simulink model "pondera2"  (R2020b)
settings: Solver=ode5  StartTime=0.0  StopTime=inf  RelTol=1e-3
undefined symbols (not defined in the file): National_Instruments, PCI
libraries: sldrtlib x2
settings Model: SimulationMode=external  Creator=Usuario_UMA  LastModifiedBy=alumnoic03
settings RTWCC: Description=Simulink Desktop Real-Time  SystemTargetFile=sldrt.tlc  TemplateMakefile=sldrt.tmf  RTWCompilerOptimization=on
settings CodeAppCC: MaxIdLength=95
settings SimulinkDesktopRealTimeCC: TargetPreCompLibLocation=C:\Program Files\MATLAB\R2020\toolbox\sldrt\lib\win64

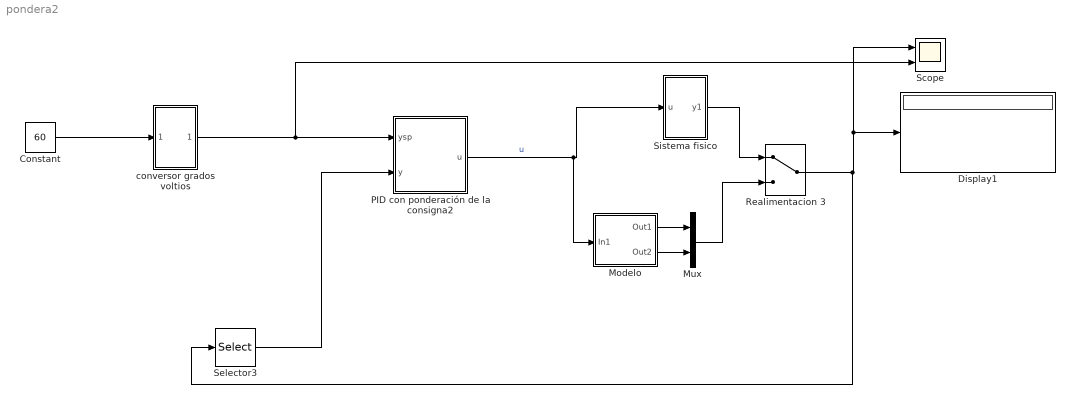
== system pondera2 ==
  Constant : Constant  Value=60
  Display1 : Display
  "Modelo " : Subsystem
  Mux : Mux  Inputs=2
  PID con ponderación de la consigna2 : Subsystem  mask{Kp=1.96, Ti=1.17, Td=0.118, b=0.85, c=0.1, N=30}
      mask prompts: Kp "Ganancia Proporcional (Kp)"; Ti "Tiempo Integral (Ti) [s]"; Td "Tiempo Derivativo (Td) [s]"; b "Peso Error Proporcional (b)"; c "Peso Error Derivativo (c)"; N "Filtro Derivativo (N) [rad/s]"
  Realimentacion 3 : ManualSwitch
  Scope : Scope  NumInputPorts=2
  Selector3 : Selector  InputPortWidth=2  IndexOptions=Index vector (dialog)  Indices=[1]  OutputSizes=1
  Sistema fisico : Subsystem
  "conversor grados voltios " : Subsystem  mask{a=4.95, b=0}
  wires:
  Constant/1 -> "conversor grados voltios "/1(In1)
  "conversor grados voltios "/1(Out1) -> PID con ponderación de la consigna2/1(ysp), Scope/2
  Selector3/1 -> PID con ponderación de la consigna2/2(y)
  PID con ponderación de la consigna2/1(u) -> "Modelo "/1(In1), Sistema fisico/1(u)  "u"
  "Modelo "/2(Out2) -> Mux/2
  "Modelo "/1(Out1) -> Mux/1
  Sistema fisico/1(y1) -> Realimentacion 3/1
  Mux/1 -> Realimentacion 3/2
  Realimentacion 3/1 -> Selector3/1, Display1/1, Scope/1

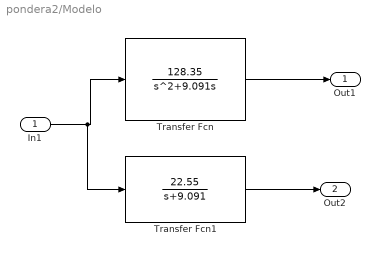
== system pondera2/Modelo  ==
  In1 : Inport
  Transfer Fcn : TransferFcn  Numerator=[128.35]  Denominator=[1 9.091 0]
  Transfer Fcn1 : TransferFcn  Numerator=[22.55]  Denominator=[1 9.091]
  Out1 : Outport
  Out2 : Outport  Port=2
  wires:
  In1/1 -> Transfer Fcn1/1, Transfer Fcn/1
  Transfer Fcn/1 -> Out1/1
  Transfer Fcn1/1 -> Out2/1

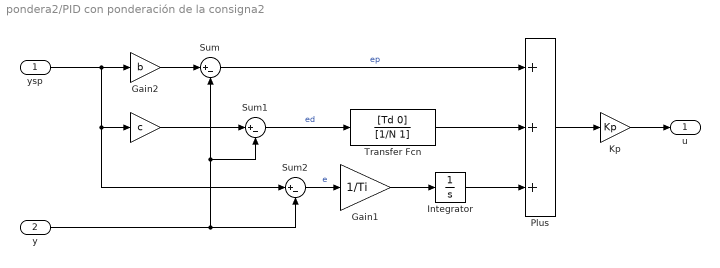
== system pondera2/PID con ponderación de la consigna2 ==
  ysp : Inport
  y : Inport  Port=2
  " " : Gain  Gain=c
  Gain1 : Gain  Gain=1/Ti
  Gain2 : Gain  Gain=b
  Integrator : Integrator
  Kp : Gain  Gain=Kp
  Plus : Sum  Inputs=+++
  Sum : Sum  Inputs=|+-
  Sum1 : Sum  Inputs=|+-
  Sum2 : Sum  Inputs=|+-
  Transfer Fcn : TransferFcn  Numerator=[Td 0]  Denominator=[1/N 1]
  u : Outport  VectorParamsAs1DForOutWhenUnconnected=off
  wires:
  Plus/1 -> Kp/1
  Kp/1 -> u/1
  Gain1/1 -> Integrator/1
  Integrator/1 -> Plus/3
  Transfer Fcn/1 -> Plus/2
  ysp/1 -> Sum2/1, " "/1, Gain2/1
  Gain2/1 -> Sum/1
  Sum/1 -> Plus/1  "ep"
  " "/1 -> Sum1/1
  Sum2/1 -> Gain1/1  "e"
  Sum1/1 -> Transfer Fcn/1  "ed"
  y/1 -> Sum/2, Sum1/2, Sum2/2

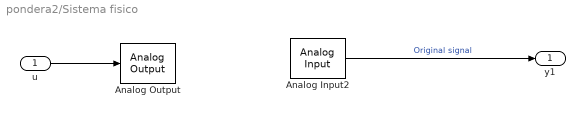
== system pondera2/Sistema fisico ==
  u : Inport
  Analog Input2 : sldrtlib/Analog Input  SampleTime=0.001  MaxMissedTicks=10  ShowMissedTicks=off  YieldWhenWaiting=off  DrvName=National_Instruments/PCI-6014  DrvAddress=4294967295  DrvOptions=[2 0 0 0 0 0]  Channels=[1,2]  RangeMode=1  VoltRange=1  DataType=1
      settings: AttributesFormatString=National Instruments\nPCI-6014 [auto]
  Analog Output : sldrtlib/Analog Output  SampleTime=0.001  MaxMissedTicks=10  ShowMissedTicks=off  YieldWhenWaiting=off  DrvName=National_Instruments/PCI-6014  DrvAddress=4294967295  DrvOptions=[2 0 0 0 0 0]  Channels=1  RangeMode=1  VoltRange=1  InitialValue=[]  FinalValue=[]
      settings: AttributesFormatString=National Instruments\nPCI-6014 [auto]
  y1 : Outport
  wires:
  u/1 -> Analog Output/1
  Analog Input2/1 -> y1/1  "Original signal"

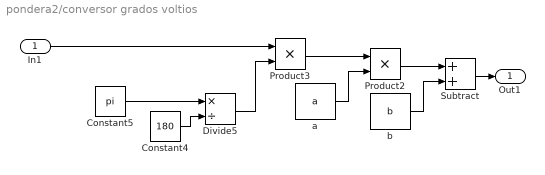
== system pondera2/conversor grados voltios  ==
  In1 : Inport
  Constant4 : Constant  Value=180
  Constant5 : Constant  Value=pi
  Divide5 : Product  Inputs=*/
  Product2 : Product
  Product3 : Product
  Subtract : Sum
  a : Constant  Value=a
  b : Constant  Value=b
  Out1 : Outport
  wires:
  b/1 -> Subtract/2
  Product3/1 -> Product2/1
  Constant4/1 -> Divide5/2
  In1/1 -> Product3/1
  Product2/1 -> Subtract/1
  a/1 -> Product2/2
  Constant5/1 -> Divide5/1
  Divide5/1 -> Product3/2
  Subtract/1 -> Out1/1
